simulink model "sim_torque_control_P_PI"  (R2021b)
settings: Solver=ode1  StartTime=0.0  StopTime=60  FixedStep=0.0001  RelTol=1e-3
values from neighbouring files (symbols this model uses):
  D = 9.4e-5*Kt    (= 4.7e-06)    [motor_parameter.m]
  J = 1.94e-4*Kt    (= 9.7e-06)    [motor_parameter.m]
  kii = (J*(-Kt^2+kpo*R)*wn^2)/(Kt*(D^2+kpo^2+J^2*wn^2-2*J*kpo*wn*zeta+2*D*(kpo-J*wn*zeta)))    (= 0.394297267374)    [motor_parameter.m]
  kpi = -(D^2*R+J^2*R*wn^2+kpo*(Kt^2-2*J*R*wn*zeta)+D*(Kt^2+R*(kpo-2*J*wn*zeta))/(Kt*(D^2+kpo^2+J^2*wn^2-2*J*kpo*wn*zeta+2*D*(kpo-J*wn*zeta))))    (= 0.0794485412984)    [motor_parameter.m]
  kpo = 10    [motor_parameter.m]
  Kt = 0.05    [motor_parameter.m]
  R = 14.3    [motor_parameter.m]
  Tc = 0.053*Kt    (= 0.00265)    [motor_parameter.m]
settings Model: Creator=ASUS  LastModifiedBy=ASUS

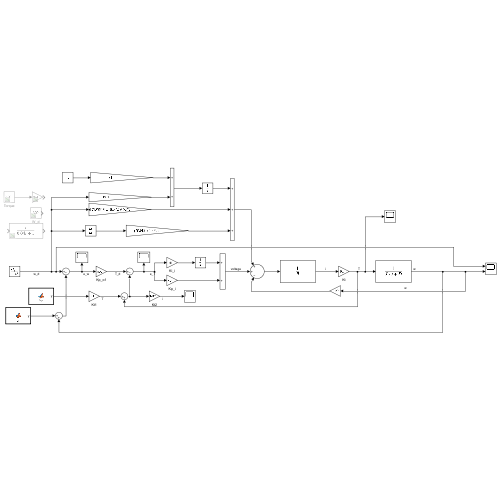
[thumbnail: Simulink's stored preview of the top-level diagram]
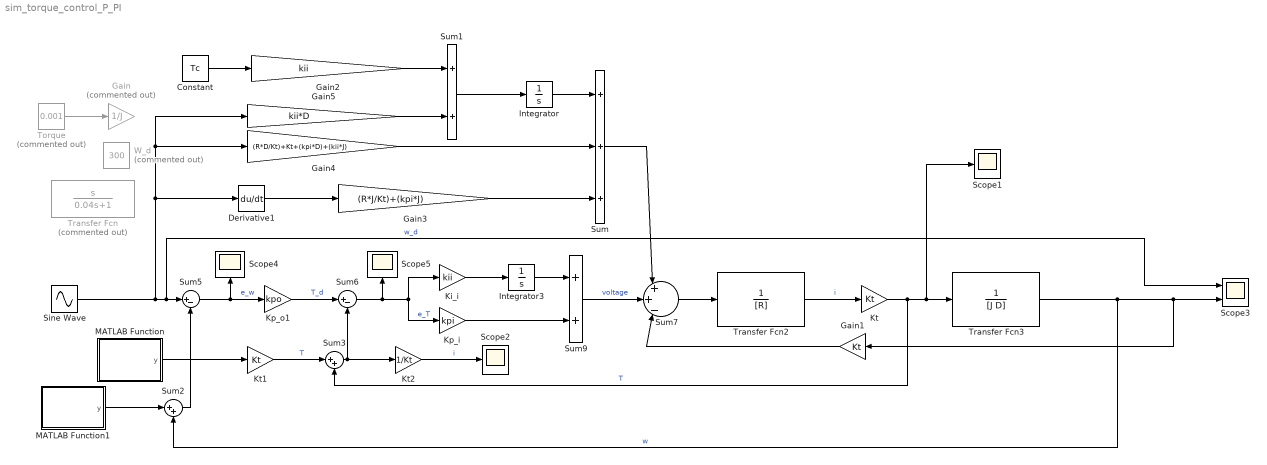
== system sim_torque_control_P_PI ==
  Constant : Constant  Value=Tc
  Derivative1 : Derivative
  Gain : Gain  Commented=on  Gain=1/J
  Gain1 : Gain  Gain=Kt
  Gain2 : Gain  Gain=kii
  Gain3 : Gain  Gain=(R*J/Kt)+(kpi*J)
  Gain4 : Gain  Gain=(R*D/Kt)+Kt+(kpi*D)+(kii*J)
  Gain5 : Gain  Gain=kii*D
  Integrator : Integrator
  Integrator3 : Integrator
  Ki_i : Gain  Gain=kii
  Kp_i : Gain  Gain=kpi
  Kp_o1 : Gain  Gain=kpo
  Kt : Gain  Gain=Kt
  Kt1 : Gain  Gain=Kt
  Kt2 : Gain  Gain=1/Kt
  MATLAB Function : MATLAB Function  TreatAsAtomicUnit=on
  MATLAB Function1 : MATLAB Function  TreatAsAtomicUnit=on
  Scope{1..2,4..5} (4 alike) : Scope
  Scope3 : Scope  NumInputPorts=2
  Sine Wave : Sin  Amplitude=150  Frequency=2*pi*0.4  SampleTime=0
  Sum : Sum  Inputs=+++
  Sum1 : Sum
  Sum2 : Sum  Inputs=|++
  Sum3 : Sum  Inputs=|++
  Sum5 : Sum  Inputs=|+-
  Sum6 : Sum  Inputs=|+-
  Sum7 : Sum  Inputs=|+|+|-|
  Sum9 : Sum
  Torque : Constant  Commented=on  Value=0.001
  Transfer Fcn : TransferFcn  Commented=on  Numerator=[1 0]  Denominator=[0.04 1]
  Transfer Fcn2 : TransferFcn  Denominator=[R]
  Transfer Fcn3 : TransferFcn  Denominator=[J D]
  W_d : Constant  Commented=on  Value=300
  wires:
  Transfer Fcn2/1 -> Kt/1  "i"
  Sum9/1 -> Sum7/2  "voltage"
  Gain1/1 -> Sum7/3
  Sum5/1 -> Kp_o1/1, Scope4/1  "e_w"
  Transfer Fcn3/1 -> Sum2/2, Scope3/2, Gain1/1  "w"
  Sum6/1 -> Ki_i/1, Kp_i/1, Scope5/1  "e_T"
  Kp_i/1 -> Sum9/2
  Kp_o1/1 -> Sum6/1  "T_d"
  Kt/1 -> Sum3/2, Scope1/1, Transfer Fcn3/1  "T"
  Ki_i/1 -> Integrator3/1
  Integrator3/1 -> Sum9/1
  Sum7/1 -> Transfer Fcn2/1
  Sine Wave/1 -> Derivative1/1, Gain4/1, Gain5/1, Scope3/1, Sum5/1  "w_d"
  Torque/1 -> Gain/1
  Constant/1 -> Gain2/1
  Gain2/1 -> Sum1/1
  Gain5/1 -> Sum1/2
  Sum1/1 -> Integrator/1
  Integrator/1 -> Sum/1
  Derivative1/1 -> Gain3/1
  Gain4/1 -> Sum/2
  Sum/1 -> Sum7/1
  Gain3/1 -> Sum/3
  Sum3/1 -> Kt2/1, Sum6/2
  MATLAB Function/1(y) -> Kt1/1
  Kt1/1 -> Sum3/1  "T"
  Sum2/1 -> Sum5/2
  MATLAB Function1/1(y) -> Sum2/1
  Kt2/1 -> Scope2/1  "i"

== matlab function sim_torque_control_P_PI/MATLAB Function ==
  data: y output
function y = fcn()
sigma = 0.1;
y = sigma*randn;

== matlab function sim_torque_control_P_PI/MATLAB Function1 ==
  data: y output
function y = fcn()
sigma = 2;
y = sigma*randn;
